simulink model "reglertest1"  (Simulink 7.4)
settings: Solver=ode45  StartTime=0.0  StopTime=1000  MaxStep=0.01  RelTol=1e-3
values from neighbouring files (symbols this model uses):
  KD = polyCOGx    [automatic_controller_2_NOPDT.m]    (also in automatic_controller_2_NOPDT_dycops.m; automatic_controller_NOPDT.m; manual_controller_NOPDT.m = KDa; stable_regions_PID5.m = optimalpolyCOGx)
  KI = polyCOGy    [automatic_controller_2_NOPDT.m]    (also in automatic_controller_2_NOPDT_dycops.m; automatic_controller_NOPDT.m; manual_controller_NOPDT.m = KIa; stable_regions_PID5.m = optimalpolyCOGy)
  KP = KPAmax    [automatic_controller_2_NOPDT.m]    (also in automatic_controller_2_NOPDT_dycops.m; automatic_controller_NOPDT.m = 0.05*KPmax; calc_max_polytope.m = KPvec(i); calc_max_polytope_NO.m = KPvec(i))
  L1 = get(Gref1,'OutputDelay')    [automatic_controller_2_NOPDT.m]    (also in automatic_controller_2_NOPDT_dycops.m)
  L2 = get(Gref2,'OutputDelay')+10    [automatic_controller_2_NOPDT.m]    (also in automatic_controller_2_NOPDT_dycops.m = get(Gref1,'OutputDelay'))
undefined symbols (not defined in the file or in its folder): Ds1, Ds2, Ns1, Ns2
libraries: simulink x6
settings Model: Creator=sle  LastModifiedBy=sle

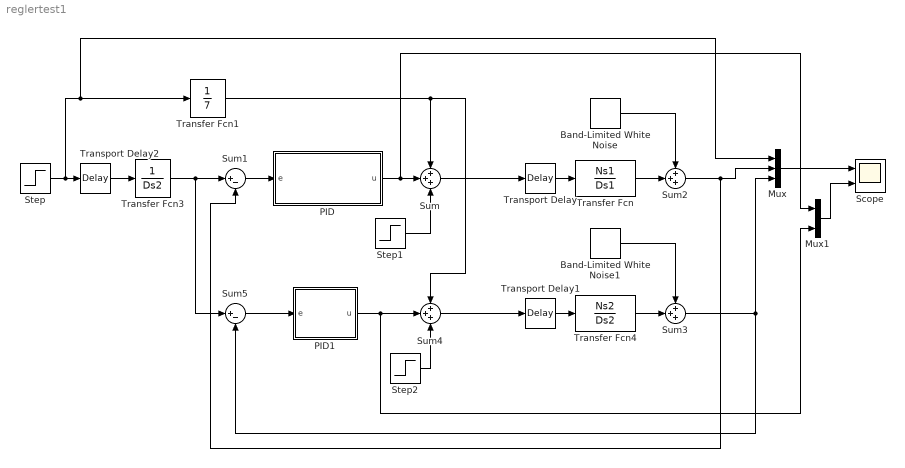
== system reglertest1 ==
  Band-Limited White Noise : simulink/Sources/Band-Limited White Noise  SystemSampleTime=-1  Cov=[0.00001]  Ts=0.1  seed=[22224]
  Band-Limited White Noise1 : simulink/Sources/Band-Limited White Noise  SystemSampleTime=-1  Cov=[0.00001]  Ts=0.1  seed=[23341]
  Mux : Mux  Inputs=3
  Mux1 : Mux  Inputs=2
  PID : Subsystem  mask{KP=KP, KI=KI, KD=KD, Tf=10, OG=900, UG=-900}
      mask prompts: Tf "Filterzeitkonstante Tf"; OG "AntiWindup Obergrenze"; UG "AntiWindup Untergrenze"
      mask init:
      | KDt=round(100*KD)/100;
      | KIt=round(100*KI)/100;
      | KPt=round(100*KP)/100;
      mask Display: dpoly([KDt KPt KIt],[Tf 1 0])
  PID1 : Subsystem  mask{KP=KP, KI=KI, KD=KD, Tf=10, OG=900, UG=-900}
      mask prompts: Tf "Filterzeitkonstante Tf"; OG "AntiWindup Obergrenze"; UG "AntiWindup Untergrenze"
  Scope : Scope  NumInputPorts=2
      settings: YMin=-0.25~-0.025  YMax=1.75~0.275
  Step : Step  Time=10  SampleTime=0
  Step1 : Step  Time=500  After=0.1  SampleTime=0
  Step2 : Step  Time=500  After=0.1  SampleTime=0
  Sum{,2..4} (4 alike) : Sum  Inputs=+++  OutDataType=fixdt(1, 16)  OutScaling=2^0
  Sum1 : Sum  Inputs=|+-  OutDataType=fixdt(1, 16)  OutScaling=2^0
  Sum5 : Sum  Inputs=|+-  OutDataType=fixdt(1, 16)  OutScaling=2^0
  Transfer Fcn : TransferFcn  Numerator=Ns1  Denominator=Ds1
  Transfer Fcn1 : TransferFcn  Numerator=1  Denominator=7
  Transfer Fcn3 : TransferFcn  Numerator=1  Denominator=Ds2
  Transfer Fcn4 : TransferFcn  Numerator=Ns2  Denominator=Ds2
  Transport Delay : TransportDelay  DelayTime=L1
  Transport Delay1 : TransportDelay  DelayTime=L2
  Transport Delay2 : TransportDelay  DelayTime=L2
  wires:
  Transport Delay/1 -> Transfer Fcn/1
  Sum/1 -> Transport Delay/1
  PID/1(u) -> Sum/2, Mux1/1
  Step/1 -> Mux/1, Transfer Fcn1/1, Transport Delay2/1
  Mux/1 -> Scope/1
  Step1/1 -> Sum/3
  Sum1/1 -> PID/1(e)
  Transfer Fcn/1 -> Sum2/2
  Sum2/1 -> Mux/2, Sum1/2
  Band-Limited White Noise/1 -> Sum2/1
  Transport Delay1/1 -> Transfer Fcn4/1
  Transfer Fcn4/1 -> Sum3/2
  Band-Limited White Noise1/1 -> Sum3/1
  Sum3/1 -> Mux/3, Sum5/2
  PID1/1(u) -> Sum4/2, Mux1/2
  Step2/1 -> Sum4/3
  Sum5/1 -> PID1/1(e)
  Sum4/1 -> Transport Delay1/1
  Mux1/1 -> Scope/2
  Transfer Fcn3/1 -> Sum1/1, Sum5/1
  Transfer Fcn1/1 -> Sum/1, Sum4/1
  Transport Delay2/1 -> Transfer Fcn3/1

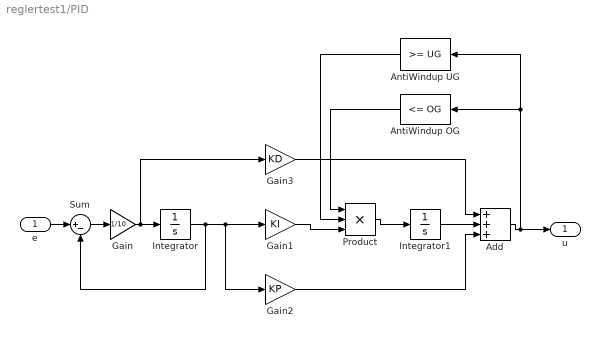
== system reglertest1/PID ==
  e : Inport  OutDataType=fixdt(1, 16)  OutScaling=2^0
  Add : Sum  Inputs=+++  OutDataType=fixdt(1, 16)  OutScaling=2^-10
  AntiWindup OG : simulink/Logic and Bit Operations/Compare To Constant  SystemSampleTime=-1  relop=<=  const=OG  LogicOutDataTypeMode=uint8  ZeroCross=off
  AntiWindup UG : simulink/Logic and Bit Operations/Compare To Constant  SystemSampleTime=-1  relop=>=  const=UG  LogicOutDataTypeMode=uint8  ZeroCross=off
  Gain : Gain  Gain=1/10  ParameterDataType=fixdt(1, 16)  ParameterScaling=2^0  OutDataType=fixdt(1, 16)  OutScaling=2^0
  Gain1 : Gain  Gain=KI  ParameterDataType=fixdt(1, 16)  ParameterScaling=2^0  OutDataType=fixdt(1, 16)  OutScaling=2^0
  Gain2 : Gain  Gain=KP  ParameterDataType=fixdt(1, 16)  ParameterScaling=2^0  OutDataType=fixdt(1, 16)  OutScaling=2^0
  Gain3 : Gain  Gain=KD  ParameterDataType=fixdt(1, 16)  ParameterScaling=2^0  OutDataType=fixdt(1, 16)  OutScaling=2^0
  Integrator : Integrator
  Integrator1 : Integrator
  Product : Product  Inputs=3  OutDataTypeMode=double  OutDataType=fixdt(1, 16)  OutScaling=2^0  OutDataTypeStr=double  RndMeth=Zero
  Sum : Sum  Inputs=|+-  OutDataType=fixdt(1, 16)  OutScaling=2^0
  u : Outport  OutDataType=fixdt(1, 16)  OutScaling=2^0
  wires:
  Add/1 -> u/1, AntiWindup UG/1, AntiWindup OG/1
  e/1 -> Sum/1
  Sum/1 -> Gain/1
  Integrator/1 -> Gain1/1, Gain2/1, Sum/2
  Product/1 -> Integrator1/1
  Integrator1/1 -> Add/2
  Gain2/1 -> Add/3
  Gain3/1 -> Add/1
  Gain1/1 -> Product/3
  AntiWindup UG/1 -> Product/2
  AntiWindup OG/1 -> Product/1
  Gain/1 -> Integrator/1, Gain3/1

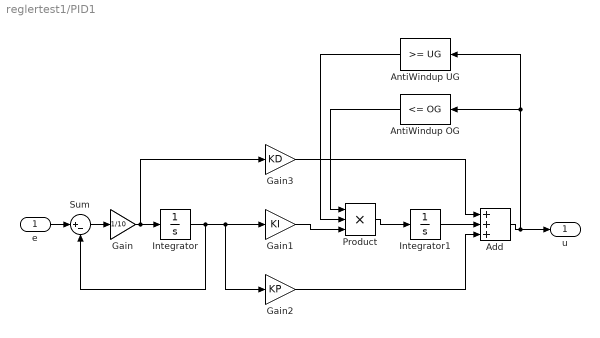
== system reglertest1/PID1 ==
  e : Inport  OutDataType=fixdt(1, 16)  OutScaling=2^0
  Add : Sum  Inputs=+++  OutDataType=fixdt(1, 16)  OutScaling=2^-10
  AntiWindup OG : simulink/Logic and Bit Operations/Compare To Constant  SystemSampleTime=-1  relop=<=  const=OG  LogicOutDataTypeMode=uint8  ZeroCross=off
  AntiWindup UG : simulink/Logic and Bit Operations/Compare To Constant  SystemSampleTime=-1  relop=>=  const=UG  LogicOutDataTypeMode=uint8  ZeroCross=off
  Gain : Gain  Gain=1/10  ParameterDataType=fixdt(1, 16)  ParameterScaling=2^0  OutDataType=fixdt(1, 16)  OutScaling=2^0
  Gain1 : Gain  Gain=KI  ParameterDataType=fixdt(1, 16)  ParameterScaling=2^0  OutDataType=fixdt(1, 16)  OutScaling=2^0
  Gain2 : Gain  Gain=KP  ParameterDataType=fixdt(1, 16)  ParameterScaling=2^0  OutDataType=fixdt(1, 16)  OutScaling=2^0
  Gain3 : Gain  Gain=KD  ParameterDataType=fixdt(1, 16)  ParameterScaling=2^0  OutDataType=fixdt(1, 16)  OutScaling=2^0
  Integrator : Integrator
  Integrator1 : Integrator
  Product : Product  Inputs=3  OutDataTypeMode=double  OutDataType=fixdt(1, 16)  OutScaling=2^0  OutDataTypeStr=double  RndMeth=Zero
  Sum : Sum  Inputs=|+-  OutDataType=fixdt(1, 16)  OutScaling=2^0
  u : Outport  OutDataType=fixdt(1, 16)  OutScaling=2^0
  wires:
  Gain/1 -> Gain3/1, Integrator/1
  AntiWindup OG/1 -> Product/1
  AntiWindup UG/1 -> Product/2
  Gain1/1 -> Product/3
  Gain3/1 -> Add/1
  Gain2/1 -> Add/3
  Integrator1/1 -> Add/2
  Product/1 -> Integrator1/1
  Integrator/1 -> Sum/2, Gain2/1, Gain1/1
  Sum/1 -> Gain/1
  e/1 -> Sum/1
  Add/1 -> AntiWindup OG/1, AntiWindup UG/1, u/1
